simulink model "PD_Controller"  (R2017b)
settings: Solver=VariableStepAuto  StartTime=0.0  StopTime=10.0  RelTol=1e-3
libraries: simulink x4
settings Model: Creator=Oguzhan  LastModifiedBy=Oguzhan

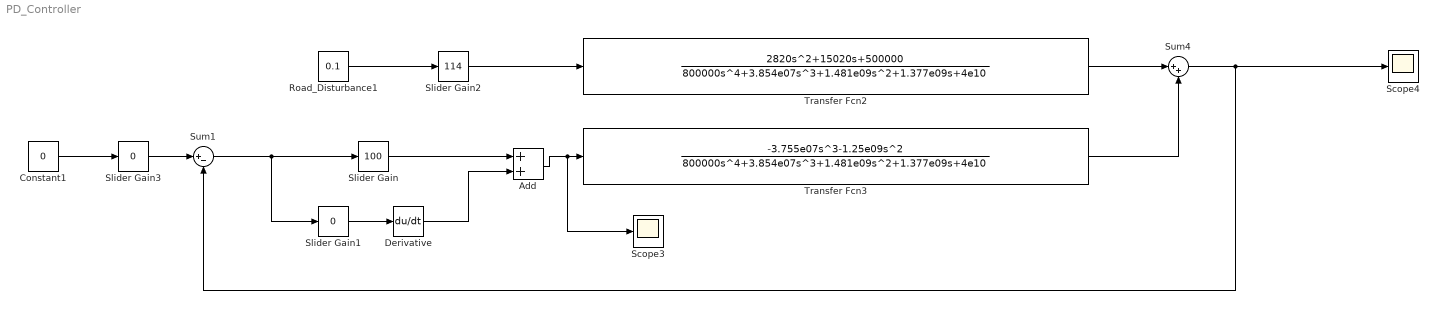
== system PD_Controller ==
  Add : Sum
  Constant1 : Constant  Value=0
  Derivative : Derivative
  Road_Disturbance1 : Constant  Value=0.1
  Scope3 : Scope
  Scope4 : Scope
  Slider Gain : simulink/Math Operations/Slider Gain  gain=100  low=1  high=2000
  Slider Gain1 : simulink/Math Operations/Slider Gain  gain=0  low=0  high=2000
  Slider Gain2 : simulink/Math Operations/Slider Gain  gain=114  low=1  high=2000
  Slider Gain3 : simulink/Math Operations/Slider Gain  gain=0  low=0  high=2000
  Sum1 : Sum  Inputs=|+-
  Sum4 : Sum  Inputs=|++
  Transfer Fcn2 : TransferFcn  Numerator=[2820 15020 500000]  Denominator=[800000 3.854e07 1.481e09 1.377e09 4e10]
  Transfer Fcn3 : TransferFcn  Numerator=[-3.755e07 -1.25e09 0 0]  Denominator=[800000 3.854e07 1.481e09 1.377e09 4e10]
  wires:
  Slider Gain1/1 -> Derivative/1
  Sum4/1 -> Scope4/1, Sum1/2
  Transfer Fcn2/1 -> Sum4/1
  Constant1/1 -> Slider Gain3/1
  Road_Disturbance1/1 -> Slider Gain2/1
  Add/1 -> Scope3/1, Transfer Fcn3/1
  Sum1/1 -> Slider Gain1/1, Slider Gain/1
  Transfer Fcn3/1 -> Sum4/2
  Slider Gain/1 -> Add/1
  Slider Gain2/1 -> Transfer Fcn2/1
  Slider Gain3/1 -> Sum1/1
  Derivative/1 -> Add/2
